simulink library "Drive_Mode_Librery"  (R2025b)
settings: Solver=VariableStepAuto  StartTime=0.0  StopTime=10.0  RelTol=1e-3

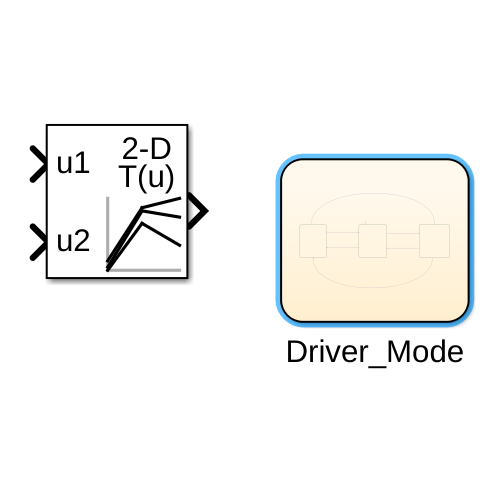
[thumbnail: Simulink's stored preview of the top-level diagram]
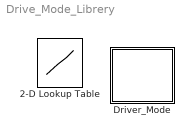
== system Drive_Mode_Librery ==
  2-D Lookup Table : Lookup_n-D  BreakpointsForDimension1=[1:3]  BreakpointsForDimension2=[1:3]  InternalRulePriority=Speed  RndMeth=Simplest
      settings: InputPortMap=u0,u1
  Driver_Mode : Stateflow chart  TreatAsAtomicUnit=on

== stateflow chart Drive_Mode_Librery/Driver_Mode ==
  state Eco
  state Normal
  state Sport
  Eco -> Sport [order 2] : [Driver_Mode_Selection == 1]
  (default) -> Normal
  Eco -> Normal [order 1] : [Driver_Mode_Selection == 2]
  Normal -> Sport [order 2] : [Driver_Mode_Selection == 1]
  Normal -> Eco [order 1] : [Driver_Mode_Selection == 0]
  Sport -> Normal [order 1] : [Driver_Mode_Selection == 2]
  Sport -> Eco [order 2] : [Driver_Mode_Selection == 0]
